simulink model "MASS_DAMPER_PID"  (R2020b)
settings: Solver=VariableStepAuto  StartTime=0.0  StopTime=T_var  RelTol=1e-3
values from neighbouring files (symbols this model uses):
  b = 10    [mass_damper_pid.m]    (also in mass_damper_pid_improved.m)
  F = 10    [mass_damper_pid.m]    (also in mass_damper_pid_improved.m = 1)
  k = 20    [mass_damper_pid.m]    (also in mass_damper_pid_improved.m)
  Kd = 300    [mass_damper_pid.m]    (also in mass_damper_pid_improved.m = 0)
  Ki = 50    [mass_damper_pid.m]    (also in mass_damper_pid_improved.m = 0)
  Kp = 500    [mass_damper_pid.m]    (also in mass_damper_pid_improved.m)
  M = 1    [mass_damper_pid.m]    (also in mass_damper_pid_improved.m)
settings Model: Creator=Raihan mahmud  LastModifiedBy=Raihan mahmud

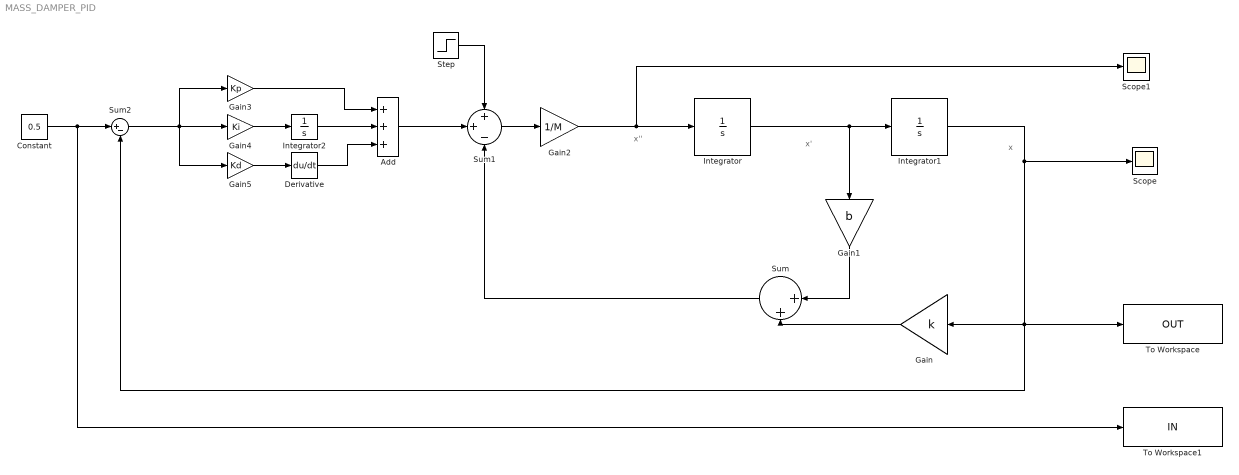
== system MASS_DAMPER_PID ==
  note: x'
  note: x''
  note: x
  Add : Sum  Inputs=+++
  Constant : Constant  Value=0.5
  Derivative : Derivative
  Gain : Gain  Gain=k
  Gain1 : Gain  Gain=b
  Gain2 : Gain  Gain=1/M
  Gain3 : Gain  Gain=Kp
  Gain4 : Gain  Gain=Ki
  Gain5 : Gain  Gain=Kd
  Integrator : Integrator
  Integrator1 : Integrator
  Integrator2 : Integrator
  Scope : Scope
  Scope1 : Scope
  Step : Step  Time=F  SampleTime=0
  Sum : Sum  Inputs=|++
  Sum1 : Sum  Inputs=++-
  Sum2 : Sum  Inputs=|+-
  To Workspace : ToWorkspace  VariableName=OUT  SaveFormat=Timeseries  SampleTime=-1
  To Workspace1 : ToWorkspace  VariableName=IN  SaveFormat=Timeseries  SampleTime=-1
  wires:
  Sum1/1 -> Gain2/1
  Integrator1/1 -> Scope/1, Gain/1, Sum2/2, To Workspace/1
  Gain/1 -> Sum/2
  Sum/1 -> Sum1/3
  Integrator/1 -> Integrator1/1, Gain1/1
  Gain1/1 -> Sum/1
  Constant/1 -> To Workspace1/1, Sum2/1
  Sum2/1 -> Gain5/1, Gain3/1, Gain4/1
  Gain4/1 -> Integrator2/1
  Gain5/1 -> Derivative/1
  Integrator2/1 -> Add/2
  Derivative/1 -> Add/3
  Gain3/1 -> Add/1
  Add/1 -> Sum1/2
  Gain2/1 -> Scope1/1, Integrator/1
  Step/1 -> Sum1/1
